simulink model "TankSystem"  (R2016b)
settings: Solver=VariableStepAuto  StartTime=0.0  StopTime=20.0  RelTol=1e-3
libraries: simulink x2
settings Model: Creator=ixohoxi  LastModifiedBy=ixohoxi

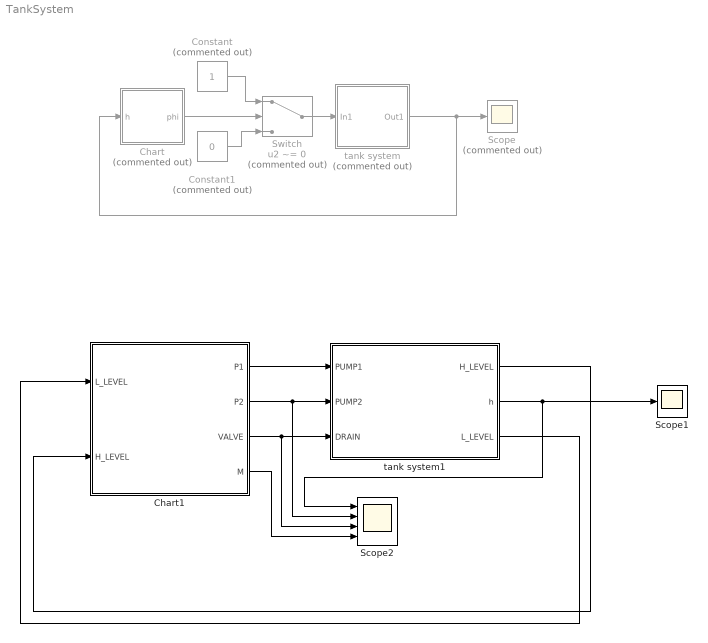
== system TankSystem ==
  Chart : Stateflow chart  Commented=on  TreatAsAtomicUnit=on
  Chart1 : Stateflow chart  TreatAsAtomicUnit=on
  Constant : Constant  Commented=on
  Constant1 : Constant  Commented=on  Value=0
  Scope : Scope  Commented=on
  Scope1 : Scope
  Scope2 : Scope  NumInputPorts=4
  Switch : Switch  Commented=on  Criteria=u2 ~= 0
  tank system : Subsystem  Commented=on  mask{a_t=1, a_h=0.1, h_0=0.5, H=1, g=9.8}
      mask prompts: a_t "tank's area"; a_h "hole's area"; h_0 "initail height"; H "maximum height"; g "gravitational acceleration"
  tank system1 : Subsystem  mask{a_t=1, a_h=0.1, h_0=0.5, H=1, g=9.8}
      mask prompts: a_t "tank's area"; a_h "hole's area"; h_0 "initail height"; H "maximum height"; g "gravitational acceleration"
  wires:
  tank system/1(Out1) -> Chart/1(h), Scope/1
  Chart/1(phi) -> Switch/2
  Switch/1 -> tank system/1(In1)
  Constant/1 -> Switch/1
  Constant1/1 -> Switch/3
  tank system1/2(h) -> Scope2/1, Scope1/1
  Chart1/1(P1) -> tank system1/1(PUMP1)
  Chart1/2(P2) -> Scope2/2, tank system1/2(PUMP2)
  Chart1/3(VALVE) -> Scope2/3, tank system1/3(DRAIN)
  tank system1/1("H_LEVEL ") -> Chart1/2(H_LEVEL)
  tank system1/3(L_LEVEL) -> Chart1/1(L_LEVEL)
  Chart1/4(M) -> Scope2/4

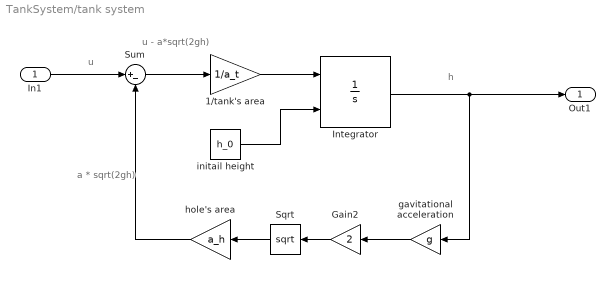
== system TankSystem/tank system ==
  note: u - a*sqrt(2gh)
  note: u
  note: a * sqrt(2gh)
  note: h
  In1 : Inport
  1/tank's area : Gain  Gain=1/a_t
  Gain2 : Gain  Gain=2
  Integrator : Integrator  InitialConditionSource=external  LimitOutput=on  UpperSaturationLimit=H  LowerSaturationLimit=0
  Sqrt : Sqrt  SaturateOnIntegerOverflow=on
  Sum : Sum  Inputs=|+-
  gavitational acceleration : Gain  Gain=g
  hole's area : Gain  Gain=a_h
  initail height : Constant  Value=h_0
  Out1 : Outport
  wires:
  Sum/1 -> 1/tank's area/1
  In1/1 -> Sum/1
  Gain2/1 -> Sqrt/1
  Sqrt/1 -> hole's area/1
  hole's area/1 -> Sum/2
  Integrator/1 -> Out1/1, gavitational acceleration/1
  initail height/1 -> Integrator/2
  gavitational acceleration/1 -> Gain2/1
  1/tank's area/1 -> Integrator/1

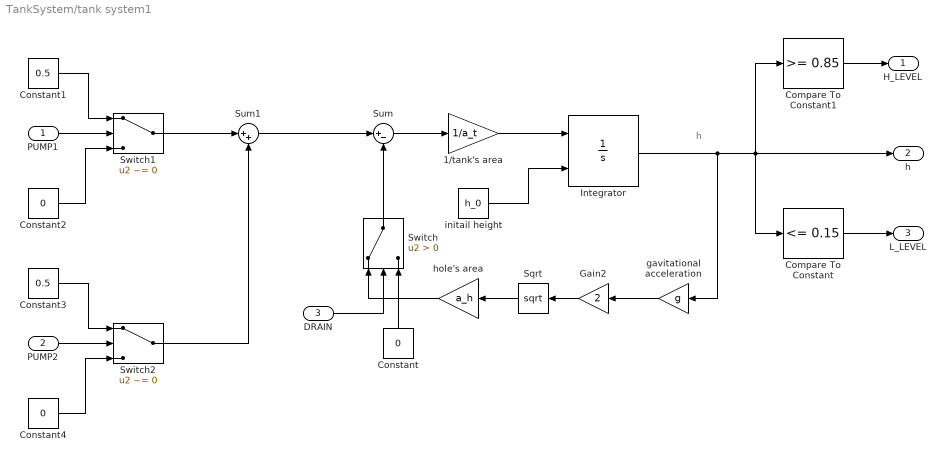
== system TankSystem/tank system1 ==
  note: h
  PUMP1 : Inport
  PUMP2 : Inport  Port=2
  DRAIN : Inport  Port=3
  1/tank's area : Gain  Gain=1/a_t
  Compare To Constant : simulink/Logic and Bit Operations/Compare To Constant  relop=<=  const=0.15  OutDataTypeStr=boolean
  Compare To Constant1 : simulink/Logic and Bit Operations/Compare To Constant  relop=>=  const=0.85  OutDataTypeStr=boolean
  Constant : Constant  Value=0
  Constant1 : Constant  Value=0.5
  Constant2 : Constant  Value=0
  Constant3 : Constant  Value=0.5
  Constant4 : Constant  Value=0
  Gain2 : Gain  Gain=2
  Integrator : Integrator  InitialConditionSource=external  LimitOutput=on  UpperSaturationLimit=H  LowerSaturationLimit=0
  Sqrt : Sqrt  SaturateOnIntegerOverflow=on
  Sum : Sum  Inputs=|+-
  Sum1 : Sum  Inputs=|++
  Switch : Switch  Criteria=u2 > Threshold
  Switch1 : Switch  Criteria=u2 ~= 0
  Switch2 : Switch  Criteria=u2 ~= 0
  gavitational acceleration : Gain  Gain=g
  hole's area : Gain  Gain=a_h
  initail height : Constant  Value=h_0
  "H_LEVEL " : Outport
  h : Outport  Port=2
  L_LEVEL : Outport  Port=3
  wires:
  Sum/1 -> 1/tank's area/1
  Gain2/1 -> Sqrt/1
  Sqrt/1 -> hole's area/1
  Integrator/1 -> gavitational acceleration/1, h/1, Compare To Constant1/1, Compare To Constant/1
  initail height/1 -> Integrator/2
  gavitational acceleration/1 -> Gain2/1
  1/tank's area/1 -> Integrator/1
  Switch/1 -> Sum/2
  hole's area/1 -> Switch/1
  Constant/1 -> Switch/3
  PUMP1/1 -> Switch1/2
  Constant1/1 -> Switch1/1
  Constant2/1 -> Switch1/3
  Constant3/1 -> Switch2/1
  Constant4/1 -> Switch2/3
  Switch2/1 -> Sum1/2
  Switch1/1 -> Sum1/1
  Sum1/1 -> Sum/1
  PUMP2/1 -> Switch2/2
  DRAIN/1 -> Switch/2
  Compare To Constant1/1 -> "H_LEVEL "/1
  Compare To Constant/1 -> L_LEVEL/1

== stateflow chart TankSystem/Chart1 ==
  settings: updateMethod=DISCRETE  sampleTime=0.01
  state FILL
  state DRAIN
  state MIX
  DRAIN -> FILL : [L_LEVEL]
      | {VALVE=false;
      | P1=true;
      | P2=true}
  (default) -> DRAIN : {M = false;
      | VALVE = true;
      | P1 = false;
      | P2 = false;
      | c =0}
  FILL -> MIX : [H_LEVEL]
      | {M=true;
      | P1=false;
      | P2=false;
      | c=c+1}
  MIX -> DRAIN [order 1] : [c>=700]
      | {M=false;
      | VALVE=true;
      | c=0}
  MIX -> MIX [order 2] : [c<700]{c=c+1}
  data: P1 output; P2 output; VALVE output; M output; c local; phi local; L_LEVEL input; H_LEVEL input; h local

== stateflow chart TankSystem/Chart ==
  settings: updateMethod=DISCRETE  sampleTime=0.01
  state OFF
  state ON
  OFF -> ON [order 1] : [h<=0.45]{phi = true}
  (default) -> OFF : {phi = false}
  ON -> ON [order 2] : [h<0.55]{phi = true}
  OFF -> OFF [order 2] : [h>0.45]{phi = false}
  ON -> OFF [order 1] : [h>=0.55]{phi = false}
  data: h input; phi output
